simulink model "exercise13b"  (R2018b)
settings: Solver=VariableStepAuto  StartTime=0.0  StopTime=10.0  RelTol=1e-3
settings Model: Creator=Alireza  LastModifiedBy=Alireza

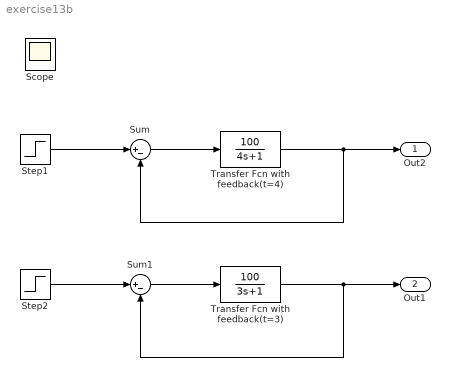
== system exercise13b ==
  Step1 : Step  SampleTime=0
  Step2 : Step  SampleTime=0
  Sum : Sum  Inputs=|+-
  Sum1 : Sum  Inputs=|+-
  Transfer Fcn with feedback(t=3) : TransferFcn  Numerator=[100]  Denominator=[3 1]
  Transfer Fcn with feedback(t=4) : TransferFcn  Numerator=[100]  Denominator=[4 1]
  Out2 : Outport
  Out1 : Outport  Port=2
  Scope : Scope
  wires:
  Transfer Fcn with feedback(t=4)/1 -> Sum/2, Out2/1
  Sum/1 -> Transfer Fcn with feedback(t=4)/1
  Step1/1 -> Sum/1
  Transfer Fcn with feedback(t=3)/1 -> Sum1/2, Out1/1
  Step2/1 -> Sum1/1
  Sum1/1 -> Transfer Fcn with feedback(t=3)/1
